simulink model "StateEstimation"  (R2024b)
settings: configuration reference "STM32H7_Config" (kept outside this file)
undefined symbols (not defined in the file): aCamberStaticFL, aCamberStaticFR, aCamberStaticRL, aCamberStaticRR, aCasterFront, AFrontalArea, aKPIFront, aRollGradient, aToeFL, aToeFR, aToeRL, aToeRR, DAirDensity, FTyreVerticalStaticFL, FTyreVerticalStaticFR, FTyreVerticalStaticRL, FTyreVerticalStaticRR, KWheelRateFront, KWheelRateRear, lFrontDistanceCG, lRearDistanceCG, lTrackWidth, lVSALLatFront, lVSALLatRear, lWheelbase, mCarMass, rAckermann, rCL, rCoP, rLLTD, zCoGHeight
libraries: simulink x4
settings Model: DataDictionary=Master_Dictionary.sldd  EnableAccessToBaseWorkspace=off  Creator=torni  LastModifiedBy=Will
settings ConfigSetRef: SourceName=STM32H7_Config

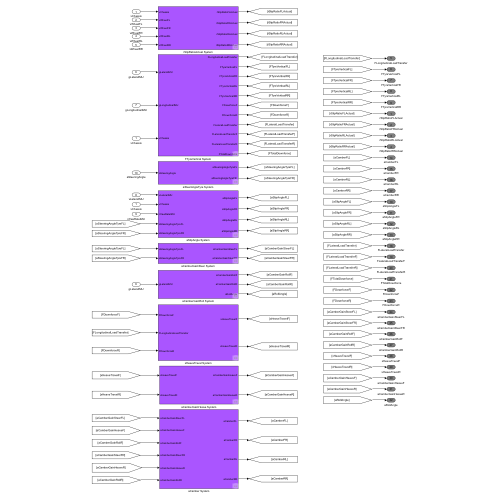
[thumbnail: Simulink's stored preview of the top-level diagram]
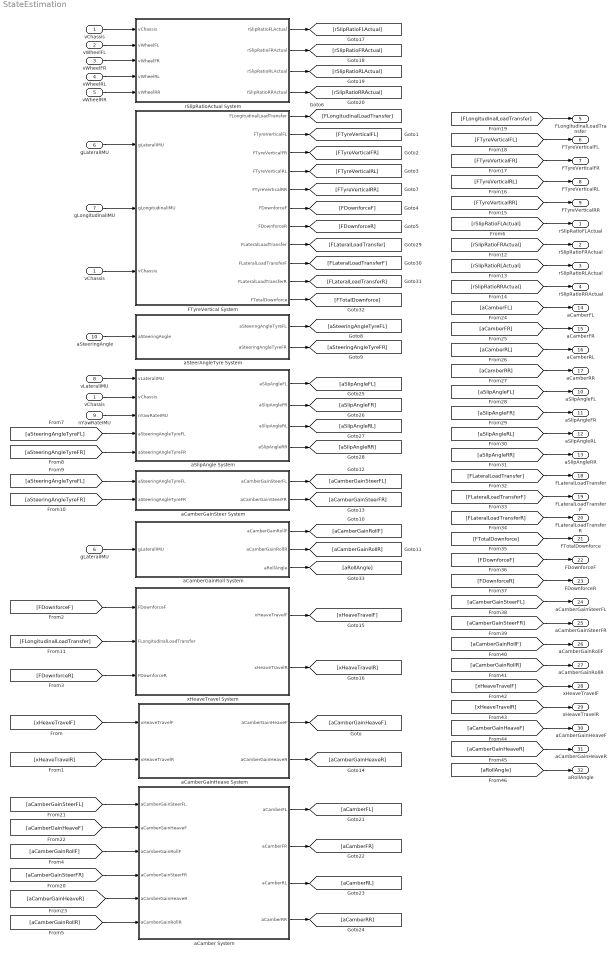
== system StateEstimation ==
  vChassis : Inport
  "vWheelFL " : Inport  Port=2
  "vWheelFR " : Inport  Port=3
  vWheelRL : Inport  Port=4
  vWheelRR : Inport  Port=5
  gLateralIMU : Inport  Port=6  OutDataTypeStr=double
  gLongitudinalIMU : Inport  Port=7  OutDataTypeStr=double
  vLateralIMU : Inport  Port=8
  nYawRateIMU : Inport  Port=9
  "aSteeringAngle " : Inport  Port=10
  FTyreVertical System : Subsystem
  aCamber System : Subsystem
  aCamberGainHeave System : Subsystem
  aCamberGainRoll System : Subsystem
  aCamberGainSteer System : Subsystem
  aSlipAngle System : Subsystem
  aSteerAngleTyre System : Subsystem
  "gLateralIMU " : InportShadow  Port=6  OutDataTypeStr=double
  rSlipRatioActual System : Subsystem
  "vChassis " : InportShadow
  "vChassis " : InportShadow
  xHeaveTravel System : Subsystem
  rSlipRatioFLActual : Outport  VectorParamsAs1DForOutWhenUnconnected=off
  rSlipRatioFRActual : Outport  Port=2  VectorParamsAs1DForOutWhenUnconnected=off
  rSlipRatioRLActual : Outport  Port=3  VectorParamsAs1DForOutWhenUnconnected=off
  rSlipRatioRRActual : Outport  Port=4  VectorParamsAs1DForOutWhenUnconnected=off
  FLongitudinalLoadTransfer : Outport  Port=5  OutDataTypeStr=double  VectorParamsAs1DForOutWhenUnconnected=off
  FTyreVerticalFL : Outport  Port=6  OutDataTypeStr=double  VectorParamsAs1DForOutWhenUnconnected=off
  FTyreVerticalFR : Outport  Port=7  OutDataTypeStr=double  VectorParamsAs1DForOutWhenUnconnected=off
  FTyreVerticalRL : Outport  Port=8  OutDataTypeStr=double  VectorParamsAs1DForOutWhenUnconnected=off
  FTyreVerticalRR : Outport  Port=9  OutDataTypeStr=double  VectorParamsAs1DForOutWhenUnconnected=off
  aSlipAngleFL : Outport  Port=10  VectorParamsAs1DForOutWhenUnconnected=off
  aSlipAngleFR : Outport  Port=11  VectorParamsAs1DForOutWhenUnconnected=off
  aSlipAngleRL : Outport  Port=12  VectorParamsAs1DForOutWhenUnconnected=off
  aSlipAngleRR : Outport  Port=13  VectorParamsAs1DForOutWhenUnconnected=off
  "aCamberFL " : Outport  Port=14  VectorParamsAs1DForOutWhenUnconnected=off
  aCamberFR : Outport  Port=15  VectorParamsAs1DForOutWhenUnconnected=off
  aCamberRL : Outport  Port=16  VectorParamsAs1DForOutWhenUnconnected=off
  aCamberRR : Outport  Port=17  VectorParamsAs1DForOutWhenUnconnected=off
  FLateralLoadTransfer : Outport  Port=18  OutDataTypeStr=double  VectorParamsAs1DForOutWhenUnconnected=off
  FLateralLoadTransferF : Outport  Port=19  OutDataTypeStr=double  VectorParamsAs1DForOutWhenUnconnected=off
  FLateralLoadTransferR : Outport  Port=20  OutDataTypeStr=double  VectorParamsAs1DForOutWhenUnconnected=off
  FTotalDownforce : Outport  Port=21  OutDataTypeStr=double  VectorParamsAs1DForOutWhenUnconnected=off
  FDownforceF : Outport  Port=22  OutDataTypeStr=double  VectorParamsAs1DForOutWhenUnconnected=off
  FDownforceR : Outport  Port=23  OutDataTypeStr=double  VectorParamsAs1DForOutWhenUnconnected=off
  aCamberGainSteerFL : Outport  Port=24  OutDataTypeStr=double  VectorParamsAs1DForOutWhenUnconnected=off
  aCamberGainSteerFR : Outport  Port=25  OutDataTypeStr=double  VectorParamsAs1DForOutWhenUnconnected=off
  aCamberGainRollF : Outport  Port=26  OutDataTypeStr=double  VectorParamsAs1DForOutWhenUnconnected=off
  aCamberGainRollR : Outport  Port=27  OutDataTypeStr=double  VectorParamsAs1DForOutWhenUnconnected=off
  xHeaveTravelF : Outport  Port=28  OutDataTypeStr=double  VectorParamsAs1DForOutWhenUnconnected=off
  xHeaveTravelR : Outport  Port=29  OutDataTypeStr=double  VectorParamsAs1DForOutWhenUnconnected=off
  aCamberGainHeaveF : Outport  Port=30  OutDataTypeStr=double  VectorParamsAs1DForOutWhenUnconnected=off
  aCamberGainHeaveR : Outport  Port=31  OutDataTypeStr=double  VectorParamsAs1DForOutWhenUnconnected=off
  aRollAngle : Outport  Port=32  VectorParamsAs1DForOutWhenUnconnected=off
  wires:
  [aCamberGainHeaveR] -> aCamber System/5("aCamberGainHeaveR ")
  [aCamberGainHeaveF] -> aCamber System/2("aCamberGainHeaveF ")
  aSteerAngleTyre System/1(aSteeringAngleTyreFL) -> [aSteeringAngleTyreFL]
  FTyreVertical System/6(FDownforceF) -> [FDownforceF]
  aCamberGainRoll System/1(aCamberGainRollF) -> [aCamberGainRollF]
  [aCamberGainSteerFR] -> aCamber System/4("aCamberGainSteerFR ")
  aCamberGainSteer System/2(aCamberGainSteerFR) -> [aCamberGainSteerFR]
  [FDownforceF] -> xHeaveTravel System/1("FDownforceF ")
  [aCamberGainRollR] -> aCamber System/6("aCamberGainRollR ")
  [aCamberGainSteerFL] -> aCamber System/1("aCamberGainSteerFL ")
  aCamberGainSteer System/1(aCamberGainSteerFL) -> [aCamberGainSteerFL]
  [FDownforceR] -> xHeaveTravel System/3("FDownforceR ")
  [aSteeringAngleTyreFL] -> aCamberGainSteer System/1(aSteeringAngleTyreFL)
  [FLongitudinalLoadTransfer] -> xHeaveTravel System/2(FLongitudinalLoadTransfer)
  [FTyreVerticalFL] -> FTyreVerticalFL/1
  [FTyreVerticalRR] -> FTyreVerticalRR/1
  "vChassis "/1 -> FTyreVertical System/3(vChassis)
  nYawRateIMU/1 -> aSlipAngle System/3("nYawRateIMU ")
  [FTyreVerticalFR] -> FTyreVerticalFR/1
  gLateralIMU/1 -> FTyreVertical System/1(gLateralIMU)
  aCamberGainRoll System/2(aCamberGainRollR) -> [aCamberGainRollR]
  FTyreVertical System/5(FTyreVerticalRR) -> [FTyreVerticalRR]
  FTyreVertical System/7(FDownforceR) -> [FDownforceR]
  vLateralIMU/1 -> aSlipAngle System/1(vLateralIMU)
  [aSteeringAngleTyreFR] -> aCamberGainSteer System/2(aSteeringAngleTyreFR)
  FTyreVertical System/1(FLongitudinalLoadTransfer) -> [FLongitudinalLoadTransfer]
  FTyreVertical System/3(FTyreVerticalFR) -> [FTyreVerticalFR]
  FTyreVertical System/4(FTyreVerticalRL) -> [FTyreVerticalRL]
  [aSteeringAngleTyreFL] -> aSlipAngle System/4(aSteeringAngleTyreFL)
  "aSteeringAngle "/1 -> aSteerAngleTyre System/1("aSteeringAngle ")
  [FLongitudinalLoadTransfer] -> FLongitudinalLoadTransfer/1
  aSteerAngleTyre System/2("aSteeringAngleTyreFR ") -> [aSteeringAngleTyreFR]
  "gLateralIMU "/1 -> aCamberGainRoll System/1("gLateralIMU ")
  FTyreVertical System/2(FTyreVerticalFL) -> [FTyreVerticalFL]
  [FTyreVerticalRL] -> FTyreVerticalRL/1
  gLongitudinalIMU/1 -> FTyreVertical System/2(gLongitudinalIMU)
  [aCamberGainRollF] -> aCamber System/3("aCamberGainRollF ")
  [aSteeringAngleTyreFR] -> aSlipAngle System/5(aSteeringAngleTyreFR)
  "vChassis "/1 -> aSlipAngle System/2(vChassis)
  xHeaveTravel System/1(xHeaveTravelF) -> [xHeaveTravelF]
  xHeaveTravel System/2(xHeaveTravelR) -> [xHeaveTravelR]
  rSlipRatioActual System/4(rSlipRatioRRActual) -> [rSlipRatioRRActual]
  rSlipRatioActual System/3(rSlipRatioRLActual) -> [rSlipRatioRLActual]
  rSlipRatioActual System/2(rSlipRatioFRActual) -> [rSlipRatioFRActual]
  rSlipRatioActual System/1(rSlipRatioFLActual) -> [rSlipRatioFLActual]
  [rSlipRatioFLActual] -> rSlipRatioFLActual/1
  [rSlipRatioRRActual] -> rSlipRatioRRActual/1
  [rSlipRatioRLActual] -> rSlipRatioRLActual/1
  [rSlipRatioFRActual] -> rSlipRatioFRActual/1
  aCamber System/1("aCamberFL ") -> [aCamberFL]
  aCamber System/2(aCamberFR) -> [aCamberFR]
  aCamber System/3(aCamberRL) -> [aCamberRL]
  aCamber System/4(aCamberRR) -> [aCamberRR]
  [aCamberFL] -> "aCamberFL "/1
  [aCamberFR] -> aCamberFR/1
  [aCamberRL] -> aCamberRL/1
  [aCamberRR] -> aCamberRR/1
  aSlipAngle System/1(aSlipAngleFL) -> [aSlipAngleFL]
  aSlipAngle System/2(aSlipAngleFR) -> [aSlipAngleFR]
  aSlipAngle System/3(aSlipAngleRL) -> [aSlipAngleRL]
  aSlipAngle System/4(aSlipAngleRR) -> [aSlipAngleRR]
  [aSlipAngleFL] -> aSlipAngleFL/1
  [aSlipAngleFR] -> aSlipAngleFR/1
  [aSlipAngleRL] -> aSlipAngleRL/1
  [aSlipAngleRR] -> aSlipAngleRR/1
  aCamberGainHeave System/1(aCamberGainHeaveF) -> [aCamberGainHeaveF]
  aCamberGainHeave System/2(aCamberGainHeaveR) -> [aCamberGainHeaveR]
  [xHeaveTravelF] -> aCamberGainHeave System/1("xHeaveTravelF ")
  [xHeaveTravelR] -> aCamberGainHeave System/2(xHeaveTravelR)
  vChassis/1 -> rSlipRatioActual System/1(vChassis)
  "vWheelFL "/1 -> rSlipRatioActual System/2("vWheelFL ")
  "vWheelFR "/1 -> rSlipRatioActual System/3("vWheelFR ")
  vWheelRL/1 -> rSlipRatioActual System/4(vWheelRL)
  vWheelRR/1 -> rSlipRatioActual System/5(vWheelRR)
  [FLateralLoadTransferR] -> FLateralLoadTransferR/1
  [FLateralLoadTransfer] -> FLateralLoadTransfer/1
  FTyreVertical System/8(FLateralLoadTransfer) -> [FLateralLoadTransfer]
  FTyreVertical System/9(FLateralLoadTransferF) -> [FLateralLoadTransferF]
  FTyreVertical System/10(FLateralLoadTransferR) -> [FLateralLoadTransferR]
  FTyreVertical System/11(FTotalDownforce) -> [FTotalDownforce]
  aCamberGainRoll System/3(aRollAngle) -> [aRollAngle]
  [FLateralLoadTransferF] -> FLateralLoadTransferF/1
  [FTotalDownforce] -> FTotalDownforce/1
  [FDownforceF] -> FDownforceF/1
  [FDownforceR] -> FDownforceR/1
  [aCamberGainSteerFL] -> aCamberGainSteerFL/1
  [aCamberGainSteerFR] -> aCamberGainSteerFR/1
  [aCamberGainRollF] -> aCamberGainRollF/1
  [aCamberGainRollR] -> aCamberGainRollR/1
  [xHeaveTravelF] -> xHeaveTravelF/1
  [xHeaveTravelR] -> xHeaveTravelR/1
  [aCamberGainHeaveF] -> aCamberGainHeaveF/1
  [aCamberGainHeaveR] -> aCamberGainHeaveR/1
  [aRollAngle] -> aRollAngle/1

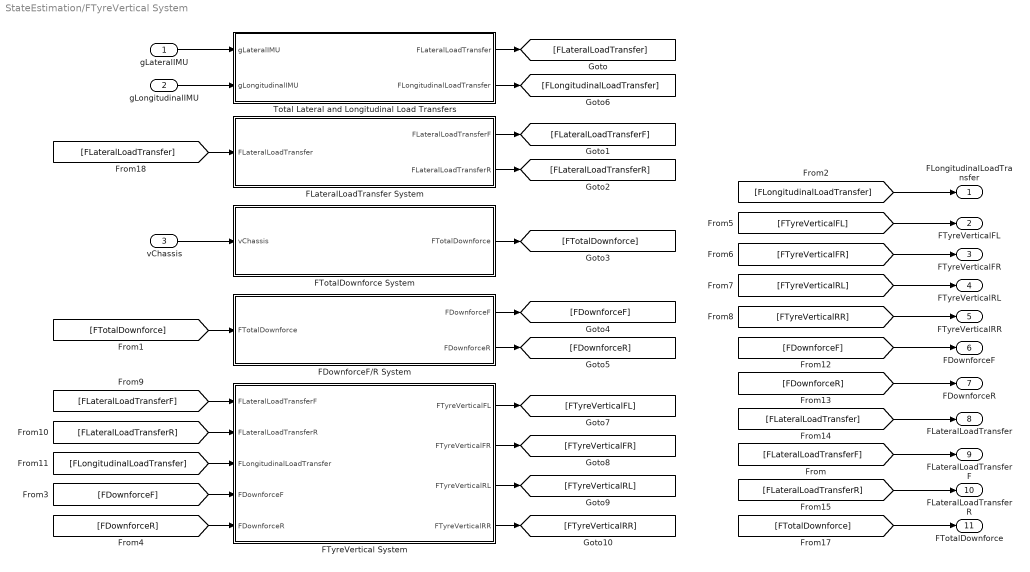
== system StateEstimation/FTyreVertical System ==
  gLateralIMU : Inport  OutDataTypeStr=double
  gLongitudinalIMU : Inport  Port=2  OutDataTypeStr=double
  vChassis : Inport  Port=3
  FDownforceF/R System : Subsystem
  FLateralLoadTransfer System : Subsystem
  FTotalDownforce System : Subsystem
  FTyreVertical System : Subsystem
  Total Lateral and Longitudinal Load Transfers : Subsystem
  FLongitudinalLoadTransfer : Outport  OutDataTypeStr=double  VectorParamsAs1DForOutWhenUnconnected=off
  FTyreVerticalFL : Outport  Port=2  OutDataTypeStr=double  VectorParamsAs1DForOutWhenUnconnected=off
  FTyreVerticalFR : Outport  Port=3  OutDataTypeStr=double  VectorParamsAs1DForOutWhenUnconnected=off
  FTyreVerticalRL : Outport  Port=4  OutDataTypeStr=double  VectorParamsAs1DForOutWhenUnconnected=off
  FTyreVerticalRR : Outport  Port=5  OutDataTypeStr=double  VectorParamsAs1DForOutWhenUnconnected=off
  FDownforceF : Outport  Port=6  OutDataTypeStr=double  VectorParamsAs1DForOutWhenUnconnected=off
  FDownforceR : Outport  Port=7  OutDataTypeStr=double  VectorParamsAs1DForOutWhenUnconnected=off
  FLateralLoadTransfer : Outport  Port=8  OutDataTypeStr=double  VectorParamsAs1DForOutWhenUnconnected=off
  FLateralLoadTransferF : Outport  Port=9  OutDataTypeStr=double  VectorParamsAs1DForOutWhenUnconnected=off
  FLateralLoadTransferR : Outport  Port=10  OutDataTypeStr=double  VectorParamsAs1DForOutWhenUnconnected=off
  FTotalDownforce : Outport  Port=11  OutDataTypeStr=double  VectorParamsAs1DForOutWhenUnconnected=off
  wires:
  [FTotalDownforce] -> FTotalDownforce/1
  FDownforceF/R System/1(FDownforceF) -> [FDownforceF]
  FLateralLoadTransfer System/1(FLateralLoadTransferF) -> [FLateralLoadTransferF]
  [FTotalDownforce] -> FDownforceF/R System/1("FTotalDownforce ")
  [FLateralLoadTransfer] -> FLateralLoadTransfer System/1(FLateralLoadTransfer)
  gLateralIMU/1 -> Total Lateral and Longitudinal Load Transfers/1(gLateralIMU)
  FLateralLoadTransfer System/2(FLateralLoadTransferR) -> [FLateralLoadTransferR]
  vChassis/1 -> FTotalDownforce System/1(vChassis)
  FTotalDownforce System/1(FTotalDownforce) -> [FTotalDownforce]
  Total Lateral and Longitudinal Load Transfers/1(FLateralLoadTransfer) -> [FLateralLoadTransfer]
  FDownforceF/R System/2(FDownforceR) -> [FDownforceR]
  [FLateralLoadTransferF] -> FTyreVertical System/1(FLateralLoadTransferF)
  [FLateralLoadTransferR] -> FTyreVertical System/2(FLateralLoadTransferR)
  [FLongitudinalLoadTransfer] -> FTyreVertical System/3("FLongitudinalLoadTransfer ")
  [FDownforceF] -> FTyreVertical System/4(FDownforceF)
  [FDownforceR] -> FTyreVertical System/5(FDownforceR)
  [FLongitudinalLoadTransfer] -> FLongitudinalLoadTransfer/1
  FTyreVertical System/1(FTyreVerticalFL) -> [FTyreVerticalFL]
  FTyreVertical System/2(FTyreVerticalFR) -> [FTyreVerticalFR]
  FTyreVertical System/3(FTyreVerticalRL) -> [FTyreVerticalRL]
  FTyreVertical System/4(FTyreVerticalRR) -> [FTyreVerticalRR]
  [FTyreVerticalFL] -> FTyreVerticalFL/1
  [FTyreVerticalFR] -> FTyreVerticalFR/1
  [FTyreVerticalRL] -> FTyreVerticalRL/1
  [FTyreVerticalRR] -> FTyreVerticalRR/1
  [FDownforceR] -> FDownforceR/1
  [FDownforceF] -> FDownforceF/1
  gLongitudinalIMU/1 -> Total Lateral and Longitudinal Load Transfers/2(gLongitudinalIMU)
  Total Lateral and Longitudinal Load Transfers/2(FLongitudinalLoadTransfer) -> [FLongitudinalLoadTransfer]
  [FLateralLoadTransfer] -> FLateralLoadTransfer/1
  [FLateralLoadTransferF] -> FLateralLoadTransferF/1
  [FLateralLoadTransferR] -> FLateralLoadTransferR/1

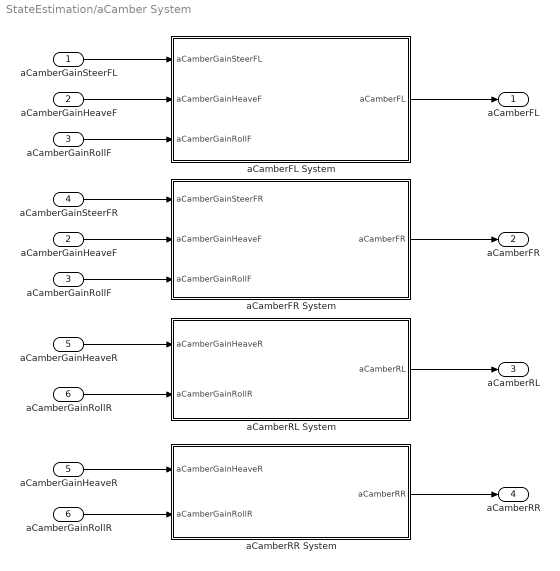
== system StateEstimation/aCamber System ==
  "aCamberGainSteerFL " : Inport
  "aCamberGainHeaveF " : Inport  Port=2
  "aCamberGainRollF " : Inport  Port=3
  "aCamberGainSteerFR " : Inport  Port=4
  "aCamberGainHeaveR " : Inport  Port=5
  "aCamberGainRollR " : Inport  Port=6
  aCamberFL System : Subsystem
  aCamberFR System : Subsystem
  "aCamberGainHeaveF " : InportShadow  Port=2
  "aCamberGainHeaveR " : InportShadow  Port=5
  "aCamberGainRollF " : InportShadow  Port=3
  "aCamberGainRollR " : InportShadow  Port=6
  aCamberRL System : Subsystem
  aCamberRR System : Subsystem
  "aCamberFL " : Outport  VectorParamsAs1DForOutWhenUnconnected=off
  aCamberFR : Outport  Port=2  VectorParamsAs1DForOutWhenUnconnected=off
  aCamberRL : Outport  Port=3  VectorParamsAs1DForOutWhenUnconnected=off
  aCamberRR : Outport  Port=4  VectorParamsAs1DForOutWhenUnconnected=off
  wires:
  "aCamberGainSteerFR "/1 -> aCamberFR System/1("aCamberGainSteerFR ")
  "aCamberGainRollR "/1 -> aCamberRR System/2("aCamberGainRollR ")
  aCamberRR System/1(aCamberRR) -> aCamberRR/1
  aCamberFL System/1("aCamberFL ") -> "aCamberFL "/1
  aCamberFR System/1(aCamberFR) -> aCamberFR/1
  "aCamberGainHeaveF "/1 -> aCamberFR System/2(aCamberGainHeaveF)
  "aCamberGainRollF "/1 -> aCamberFR System/3("aCamberGainRollF ")
  aCamberRL System/1(aCamberRL) -> aCamberRL/1
  "aCamberGainRollR "/1 -> aCamberRL System/2("aCamberGainRollR ")
  "aCamberGainHeaveR "/1 -> aCamberRL System/1("aCamberGainHeaveR ")
  "aCamberGainRollF "/1 -> aCamberFL System/3(aCamberGainRollF)
  "aCamberGainSteerFL "/1 -> aCamberFL System/1(aCamberGainSteerFL)
  "aCamberGainHeaveF "/1 -> aCamberFL System/2("aCamberGainHeaveF ")
  "aCamberGainHeaveR "/1 -> aCamberRR System/1("aCamberGainHeaveR ")

== system StateEstimation/aCamberGainHeave System ==
  note: Camber Gain Heave Angle Front = ( atan ( Heave Travel Distance Front / Virtual Swing Arm Length Lateral Front )) * (180/pi)
  note: Camber Gain Heave Angle Rear = ( atan (Heave Travel Distance Rear / Virtual Swing Arm Length Lateral Rear )) * (180/pi)
  "xHeaveTravelF " : Inport
  xHeaveTravelR : Inport  Port=2
  Constant : Constant  Value=lVSALLatFront
  Constant1 : Constant  Value=lVSALLatRear
  Demux : Demux  Outputs=2
  Divide : Product  Inputs=*/
  Gain : Gain  Gain=180/pi
  Mux : Mux  Inputs=2
  Mux1 : Mux  Inputs=2
  Trigonometric Function : Trigonometry  Operator=atan
  aCamberGainHeaveF : Outport  VectorParamsAs1DForOutWhenUnconnected=off
  aCamberGainHeaveR : Outport  Port=2  VectorParamsAs1DForOutWhenUnconnected=off
  wires:
  Trigonometric Function/1 -> Gain/1
  Divide/1 -> Trigonometric Function/1
  Mux/1 -> Divide/1
  Gain/1 -> Demux/1
  xHeaveTravelR/1 -> Mux/2
  "xHeaveTravelF "/1 -> Mux/1
  Demux/1 -> aCamberGainHeaveF/1
  Demux/2 -> aCamberGainHeaveR/1
  Constant/1 -> Mux1/1
  Mux1/1 -> Divide/2
  Constant1/1 -> Mux1/2

== system StateEstimation/aCamberGainRoll System ==
  "gLateralIMU " : Inport
  aCamberGainRoll System : Subsystem
  aRollAngle System : Subsystem
  aCamberGainRollF : Outport  VectorParamsAs1DForOutWhenUnconnected=off
  aCamberGainRollR : Outport  Port=2  VectorParamsAs1DForOutWhenUnconnected=off
  aRollAngle : Outport  Port=3  VectorParamsAs1DForOutWhenUnconnected=off
  wires:
  "gLateralIMU "/1 -> aRollAngle System/1("gLateralIMU ")
  [aRollAngle] -> aCamberGainRoll System/1(aRollAngle)
  aCamberGainRoll System/1(aCamberGainRollF) -> aCamberGainRollF/1
  aCamberGainRoll System/2("aCamberGainRollR ") -> aCamberGainRollR/1
  aRollAngle System/1("aRollAngle ") -> aRollAngle/1

== system StateEstimation/aCamberGainSteer System ==
  aSteeringAngleTyreFL : Inport
  aSteeringAngleTyreFR : Inport  Port=2
  aCamberGainSteerFL System : Subsystem
  aCamberGainSteerFR System : Subsystem
  aCamberGainSteerFL : Outport  VectorParamsAs1DForOutWhenUnconnected=off
  aCamberGainSteerFR : Outport  Port=2  VectorParamsAs1DForOutWhenUnconnected=off
  wires:
  aSteeringAngleTyreFR/1 -> aCamberGainSteerFR System/1(aSteeringAngleTyreFR)
  aSteeringAngleTyreFL/1 -> aCamberGainSteerFL System/1(aSteeringAngleTyreFL)
  aCamberGainSteerFL System/1(aCamberGainSteerFL) -> aCamberGainSteerFL/1
  aCamberGainSteerFR System/1(aCamberGainSteerFR) -> aCamberGainSteerFR/1

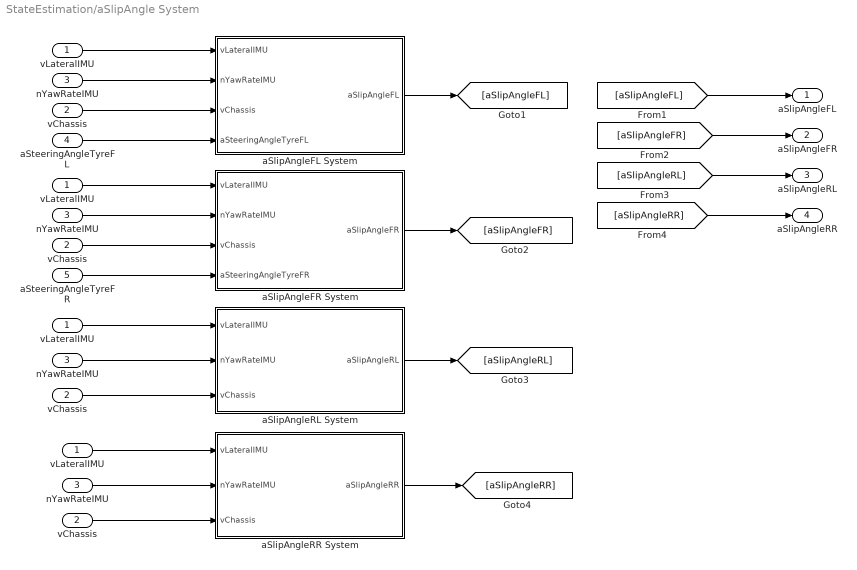
== system StateEstimation/aSlipAngle System ==
  vLateralIMU : Inport
  vChassis : Inport  Port=2
  "nYawRateIMU " : Inport  Port=3
  aSteeringAngleTyreFL : Inport  Port=4
  aSteeringAngleTyreFR : Inport  Port=5
  aSlipAngleFL System : Subsystem
  aSlipAngleFR System : Subsystem
  aSlipAngleRL System : Subsystem
  aSlipAngleRR System : Subsystem
  "nYawRateIMU " : InportShadow  Port=3
  "nYawRateIMU " : InportShadow  Port=3
  "nYawRateIMU " : InportShadow  Port=3
  "vChassis " : InportShadow  Port=2
  "vChassis " : InportShadow  Port=2
  "vChassis " : InportShadow  Port=2
  "vLateralIMU " : InportShadow
  "vLateralIMU " : InportShadow
  "vLateralIMU " : InportShadow
  aSlipAngleFL : Outport  VectorParamsAs1DForOutWhenUnconnected=off
  aSlipAngleFR : Outport  Port=2  VectorParamsAs1DForOutWhenUnconnected=off
  aSlipAngleRL : Outport  Port=3  VectorParamsAs1DForOutWhenUnconnected=off
  aSlipAngleRR : Outport  Port=4  VectorParamsAs1DForOutWhenUnconnected=off
  wires:
  aSlipAngleFR System/1(aSlipAngleFR) -> [aSlipAngleFR]
  "nYawRateIMU "/1 -> aSlipAngleFR System/2(nYawRateIMU)
  [aSlipAngleRR] -> aSlipAngleRR/1
  "nYawRateIMU "/1 -> aSlipAngleFL System/2(nYawRateIMU)
  [aSlipAngleRL] -> aSlipAngleRL/1
  vLateralIMU/1 -> aSlipAngleFL System/1("vLateralIMU ")
  [aSlipAngleFL] -> aSlipAngleFL/1
  "nYawRateIMU "/1 -> aSlipAngleRR System/2("nYawRateIMU  ")
  aSlipAngleRR System/1(aSlipAngleRR) -> [aSlipAngleRR]
  aSteeringAngleTyreFL/1 -> aSlipAngleFL System/4(aSteeringAngleTyreFL)
  "nYawRateIMU "/1 -> aSlipAngleRL System/2("nYawRateIMU ")
  aSteeringAngleTyreFR/1 -> aSlipAngleFR System/4(aSteeringAngleTyreFR)
  [aSlipAngleFR] -> aSlipAngleFR/1
  aSlipAngleFL System/1(aSlipAngleFL) -> [aSlipAngleFL]
  aSlipAngleRL System/1(aSlipAngleRL) -> [aSlipAngleRL]
  vChassis/1 -> aSlipAngleFL System/3("vChassis ")
  "vLateralIMU "/1 -> aSlipAngleFR System/1("vLateralIMU  ")
  "vLateralIMU "/1 -> aSlipAngleRL System/1("vLateralIMU   ")
  "vLateralIMU "/1 -> aSlipAngleRR System/1("vLateralIMU    ")
  "vChassis "/1 -> aSlipAngleFR System/3("vChassis  ")
  "vChassis "/1 -> aSlipAngleRR System/3("vChassis ")
  "vChassis "/1 -> aSlipAngleRL System/3("vChassis   ")

== system StateEstimation/aSteerAngleTyre System ==
  "aSteeringAngle " : Inport
  "aSteeringAngle " : InportShadow
  aSteeringAngleTyreFL System : Subsystem
  aSteeringAngleTyreFR System : Subsystem
  aSteeringAngleTyreFL : Outport  VectorParamsAs1DForOutWhenUnconnected=off
  "aSteeringAngleTyreFR " : Outport  Port=2  VectorParamsAs1DForOutWhenUnconnected=off
  wires:
  aSteeringAngleTyreFL System/1(aSteeringAngleTyreFL) -> aSteeringAngleTyreFL/1
  aSteeringAngleTyreFR System/1("aSteeringAngleTyreFR ") -> "aSteeringAngleTyreFR "/1
  "aSteeringAngle "/1 -> aSteeringAngleTyreFR System/1(aSteeringAngle)
  "aSteeringAngle "/1 -> aSteeringAngleTyreFL System/1(aSteeringAngle)

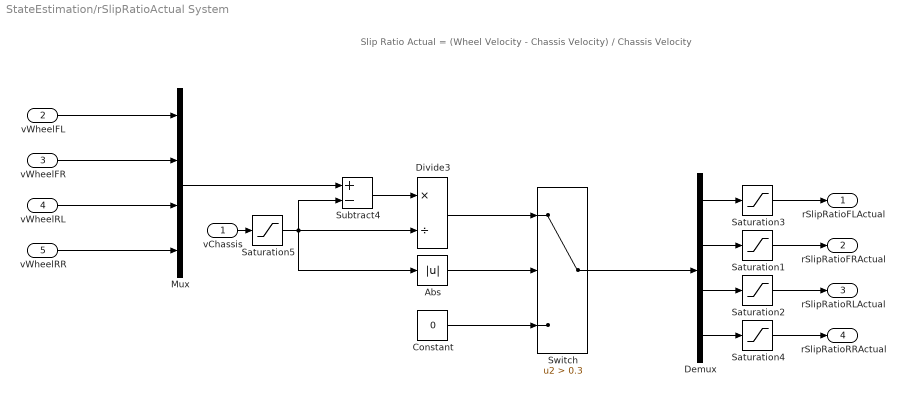
== system StateEstimation/rSlipRatioActual System ==
  note: Slip Ratio Actual = (Wheel Velocity - Chassis Velocity) / Chassis Velocity
  vChassis : Inport
  "vWheelFL " : Inport  Port=2
  "vWheelFR " : Inport  Port=3
  vWheelRL : Inport  Port=4
  vWheelRR : Inport  Port=5
  Abs : Abs  SaturateOnIntegerOverflow=off
  Constant : Constant  Value=0
  Demux : Demux
  Divide3 : Product  Inputs=*/
  Mux : Mux
  Saturation{1..4} (4 alike) : Saturate  UpperLimit=1  LowerLimit=-1
  Saturation5 : Saturate  UpperLimit=35  LowerLimit=0
  Subtract4 : Sum  Inputs=+-
  Switch : Switch  Criteria=u2 > Threshold  Threshold=0.3  SaturateOnIntegerOverflow=off  InputSameDT=off
  rSlipRatioFLActual : Outport  VectorParamsAs1DForOutWhenUnconnected=off
  rSlipRatioFRActual : Outport  Port=2  VectorParamsAs1DForOutWhenUnconnected=off
  rSlipRatioRLActual : Outport  Port=3  VectorParamsAs1DForOutWhenUnconnected=off
  rSlipRatioRRActual : Outport  Port=4  VectorParamsAs1DForOutWhenUnconnected=off
  wires:
  Demux/3 -> Saturation2/1
  Demux/2 -> Saturation1/1
  Abs/1 -> Switch/2
  Subtract4/1 -> Divide3/1
  Demux/1 -> Saturation3/1
  Demux/4 -> Saturation4/1
  Divide3/1 -> Switch/1
  Constant/1 -> Switch/3
  vWheelRR/1 -> Mux/4
  "vWheelFL "/1 -> Mux/1
  Switch/1 -> Demux/1
  vChassis/1 -> Saturation5/1
  "vWheelFR "/1 -> Mux/2
  Mux/1 -> Subtract4/1
  vWheelRL/1 -> Mux/3
  Saturation3/1 -> rSlipRatioFLActual/1
  Saturation1/1 -> rSlipRatioFRActual/1
  Saturation2/1 -> rSlipRatioRLActual/1
  Saturation4/1 -> rSlipRatioRRActual/1
  Saturation5/1 -> Abs/1, Subtract4/2, Divide3/2

== system StateEstimation/xHeaveTravel System ==
  "FDownforceF " : Inport
  FLongitudinalLoadTransfer : Inport  Port=2
  "FDownforceR " : Inport  Port=3
  "FLongitudinalLoadTransfer " : InportShadow  Port=2
  xHeaveTravelF System : Subsystem
  xHeaveTravelR System : Subsystem
  xHeaveTravelF : Outport  VectorParamsAs1DForOutWhenUnconnected=off
  xHeaveTravelR : Outport  Port=2  VectorParamsAs1DForOutWhenUnconnected=off
  wires:
  "FDownforceF "/1 -> xHeaveTravelF System/1("FDownforceF ")
  "FDownforceR "/1 -> xHeaveTravelR System/1("FDownforceR ")
  xHeaveTravelR System/1(xHeaveTravelR) -> xHeaveTravelR/1
  FLongitudinalLoadTransfer/1 -> xHeaveTravelF System/2(FLongitudinalLoadTransfer)
  xHeaveTravelF System/1(xHeaveTravelF) -> xHeaveTravelF/1
  "FLongitudinalLoadTransfer "/1 -> xHeaveTravelR System/2("FLongitudinalLoadTransfer ")

== system StateEstimation/FTyreVertical System/FDownforceF//R System ==
  note: Front Downforce = Total Downforce * CoP
      | Rear Downforce = Total Downforce * (1-CoP)
  "FTotalDownforce " : Inport  OutDataTypeStr=double
  "1 - pCoP " : Gain  Gain=1 - rCoP
  CoP : Gain  Gain=rCoP
  FDownforceF : Outport  OutDataTypeStr=double  VectorParamsAs1DForOutWhenUnconnected=off
  FDownforceR : Outport  Port=2  OutDataTypeStr=double  VectorParamsAs1DForOutWhenUnconnected=off
  wires:
  CoP/1 -> FDownforceF/1
  "FTotalDownforce "/1 -> "1 - pCoP "/1, CoP/1
  "1 - pCoP "/1 -> FDownforceR/1

== system StateEstimation/FTyreVertical System/FLateralLoadTransfer System ==
  note: Front Lateral Load Transfer = Total Lateral Load Transfer * LLTD
  note: Rear Lateral Load Transfer = Total Lateral Load Transfer * (1-LLTD)
  FLateralLoadTransfer : Inport  OutDataTypeStr=double
  1-LLTD : Gain  Gain=1 - rLLTD
  LLTD : Gain  Gain=rLLTD
  FLateralLoadTransferF : Outport  OutDataTypeStr=double  VectorParamsAs1DForOutWhenUnconnected=off
  FLateralLoadTransferR : Outport  Port=2  OutDataTypeStr=double  VectorParamsAs1DForOutWhenUnconnected=off
  wires:
  LLTD/1 -> FLateralLoadTransferF/1
  FLateralLoadTransfer/1 -> 1-LLTD/1, LLTD/1
  1-LLTD/1 -> FLateralLoadTransferR/1

== system StateEstimation/FTyreVertical System/FTotalDownforce System ==
  note: Total Downforce = 0.5 * Air Density * Chassis Velocity ^2 * Frontal area * CL
  vChassis : Inport  OutDataTypeStr=double
  " " : Gain  Gain=0.5
  Air Density : Gain  Gain=DAirDensity
  CL : Gain  Gain=rCL
  Frontal Area : Gain  Gain=AFrontalArea
  Square : Math  Operator=square  SignedPower=on
  FTotalDownforce : Outport  OutDataTypeStr=double  VectorParamsAs1DForOutWhenUnconnected=off
  wires:
  Frontal Area/1 -> CL/1
  " "/1 -> Frontal Area/1
  Air Density/1 -> " "/1
  vChassis/1 -> Square/1
  Square/1 -> Air Density/1
  CL/1 -> FTotalDownforce/1

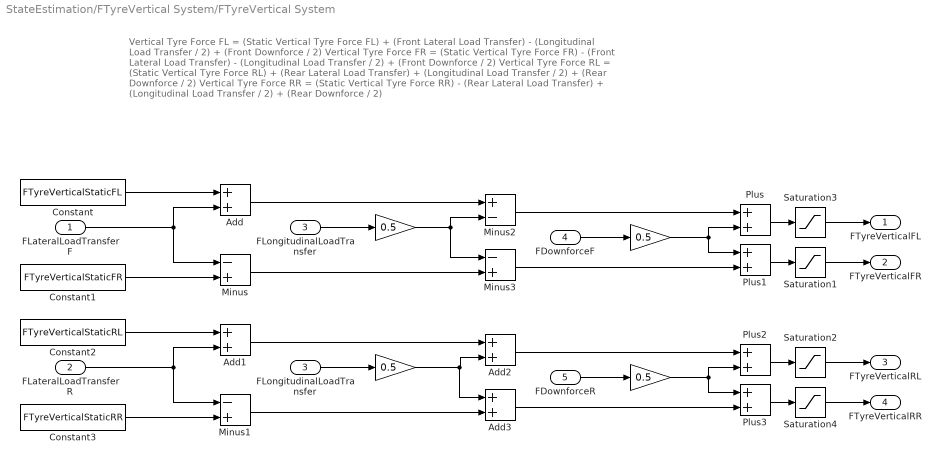
== system StateEstimation/FTyreVertical System/FTyreVertical System ==
  note: Vertical Tyre Force FL = (Static Vertical Tyre Force FL) + (Front Lateral Load Transfer) - (Longitudinal Load Transfer / 2) + (Front Downforce / 2)
      |
      | Vertical Tyre Force FR = (Static Vertical Tyre Force FR) - (Front Lateral Load Transfer) - (Longitudinal Load Transfer / 2) + (Front Downforce / 2)
      |
      | Vertical Tyre Force RL = (Static Vertical Tyre Force RL) + (Rear Lateral Load Transfer) + (Longitudinal Load Transfer / 2) + (Rear Downforce / 2)
      |
      | Vertical Tyre Force RR = (Static Vertical Tyre Force RR) - (Rear Lateral Load Transfer) + (Longitudinal Load Transfer / 2) + (Rear Downforce / 2)
  FLateralLoadTransferF : Inport
  FLateralLoadTransferR : Inport  Port=2
  "FLongitudinalLoadTransfer " : Inport  Port=3
  FDownforceF : Inport  Port=4
  FDownforceR : Inport  Port=5
   {,,,} (4 alike) : Gain  Gain=0.5
  Add{,1..3} (4 alike) : Sum
  Constant : Constant  Value=FTyreVerticalStaticFL
  Constant1 : Constant  Value=FTyreVerticalStaticFR
  Constant2 : Constant  Value=FTyreVerticalStaticRL
  Constant3 : Constant  Value=FTyreVerticalStaticRR
  "FLongitudinalLoadTransfer " : InportShadow  Port=3
  Minus : Sum  Inputs=-+
  Minus1 : Sum  Inputs=-+
  Minus2 : Sum  Inputs=+-
  Minus3 : Sum  Inputs=-+
  Plus{,1..3} (4 alike) : Sum
  Saturation{1..4} (4 alike) : Saturate  UpperLimit=2300  LowerLimit=0
  FTyreVerticalFL : Outport  OutDataTypeStr=double  VectorParamsAs1DForOutWhenUnconnected=off
  FTyreVerticalFR : Outport  Port=2  OutDataTypeStr=double  VectorParamsAs1DForOutWhenUnconnected=off
  FTyreVerticalRL : Outport  Port=3  OutDataTypeStr=double  VectorParamsAs1DForOutWhenUnconnected=off
  FTyreVerticalRR : Outport  Port=4  OutDataTypeStr=double  VectorParamsAs1DForOutWhenUnconnected=off
  wires:
  Minus/1 -> Minus3/2
  "FLongitudinalLoadTransfer "/1 -> " "/1
  FLateralLoadTransferR/1 -> Minus1/1, Add1/2
  FDownforceF/1 -> " "/1
  Minus2/1 -> Plus/1
  " "/1 -> Plus3/1, Plus2/2
  Plus3/1 -> Saturation4/1
  Add2/1 -> Plus2/1
  " "/1 -> Minus3/1, Minus2/2
  Plus2/1 -> Saturation2/1
  " "/1 -> Add3/1, Add2/2
  " "/1 -> Plus1/1, Plus/2
  Constant3/1 -> Minus1/2
  FLateralLoadTransferF/1 -> Minus/1, Add/2
  Constant2/1 -> Add1/1
  FDownforceR/1 -> " "/1
  Add/1 -> Minus2/1
  Plus1/1 -> Saturation1/1
  Constant1/1 -> Minus/2
  Add1/1 -> Add2/1
  Minus3/1 -> Plus1/2
  Minus1/1 -> Add3/2
  Add3/1 -> Plus3/2
  "FLongitudinalLoadTransfer "/1 -> " "/1
  Constant/1 -> Add/1
  Plus/1 -> Saturation3/1
  Saturation3/1 -> FTyreVerticalFL/1
  Saturation1/1 -> FTyreVerticalFR/1
  Saturation2/1 -> FTyreVerticalRL/1
  Saturation4/1 -> FTyreVerticalRR/1

== system StateEstimation/FTyreVertical System/Total Lateral and Longitudinal Load Transfers ==
  note: update values
  note: Lateral Load Transfer = (Lateral Acceleration * Mass * CoG Height) / Trackwidth
  note: Longitudinal Load Transfer = (Longitudinal Acceleration * Mass * CoG Height) / Wheelbase
  gLateralIMU : Inport  OutDataTypeStr=double
  gLongitudinalIMU : Inport  Port=2  OutDataTypeStr=double
  1/Trackwidth : Gain  Gain=1/lTrackWidth
  1/Wheelbase : Gain  Gain=1/lWheelbase
  CoG Height : Gain  Gain=zCoGHeight
  Demux : Demux  Outputs=2
  Mass : Gain  Gain=mCarMass
  Mux : Mux  Inputs=2
  FLateralLoadTransfer : Outport  OutDataTypeStr=double  VectorParamsAs1DForOutWhenUnconnected=off
  FLongitudinalLoadTransfer : Outport  Port=2  OutDataTypeStr=double  VectorParamsAs1DForOutWhenUnconnected=off
  wires:
  Mass/1 -> CoG Height/1
  Mux/1 -> Mass/1
  gLongitudinalIMU/1 -> Mux/2
  gLateralIMU/1 -> Mux/1
  Demux/2 -> 1/Wheelbase/1
  Demux/1 -> 1/Trackwidth/1
  CoG Height/1 -> Demux/1
  1/Wheelbase/1 -> FLongitudinalLoadTransfer/1
  1/Trackwidth/1 -> FLateralLoadTransfer/1

== system StateEstimation/aCamber System/aCamberFL System ==
  note: Camber Angle FL = Static Camber Angle FL + Camber Gain Steer Angle FL - Camber Gain Heave Angle Front + aCamberGainRollFront
  aCamberGainSteerFL : Inport
  "aCamberGainHeaveF " : Inport  Port=2
  aCamberGainRollF : Inport  Port=3
  Add : Sum
  Add1 : Sum
  Constant : Constant  Value=aCamberStaticFL
  Saturation3 : Saturate  UpperLimit=7  LowerLimit=-7
  Subtract : Sum  Inputs=+-
  "aCamberFL " : Outport  VectorParamsAs1DForOutWhenUnconnected=off
  wires:
  Add1/1 -> Saturation3/1
  "aCamberGainHeaveF "/1 -> Subtract/2
  Add/1 -> Subtract/1
  aCamberGainRollF/1 -> Add1/2
  aCamberGainSteerFL/1 -> Add/2
  Subtract/1 -> Add1/1
  Constant/1 -> Add/1
  Saturation3/1 -> "aCamberFL "/1

== system StateEstimation/aCamber System/aCamberFR System ==
  note: Camber Angle FR = Static Camber Angle FR + Camber Gain Steer Angle FR - Camber Gain Heave Angle Front - Camber Gain Roll Angle Front
  "aCamberGainSteerFR " : Inport
  aCamberGainHeaveF : Inport  Port=2
  "aCamberGainRollF " : Inport  Port=3
  Add : Sum
  Constant : Constant  Value=aCamberStaticFR
  Saturation3 : Saturate  UpperLimit=7  LowerLimit=-7
  Subtract : Sum  Inputs=+-
  Subtract1 : Sum  Inputs=+-
  aCamberFR : Outport  VectorParamsAs1DForOutWhenUnconnected=off
  wires:
  Subtract/1 -> Subtract1/1
  "aCamberGainRollF "/1 -> Subtract1/2
  aCamberGainHeaveF/1 -> Subtract/2
  "aCamberGainSteerFR "/1 -> Add/2
  Constant/1 -> Add/1
  Subtract1/1 -> Saturation3/1
  Add/1 -> Subtract/1
  Saturation3/1 -> aCamberFR/1

== system StateEstimation/aCamber System/aCamberRL System ==
  note: Camber Angle RL = Static Camber Angle RL - Camber Gain Heave Angle Rear + Camber Gain Roll Angle Rear
  "aCamberGainHeaveR " : Inport
  "aCamberGainRollR " : Inport  Port=2
  Add : Sum
  Constant : Constant  Value=aCamberStaticRL
  Saturation3 : Saturate  UpperLimit=7  LowerLimit=-7
  Subtract : Sum  Inputs=+-
  aCamberRL : Outport  VectorParamsAs1DForOutWhenUnconnected=off
  wires:
  "aCamberGainHeaveR "/1 -> Subtract/2
  "aCamberGainRollR "/1 -> Add/2
  Subtract/1 -> Add/1
  Add/1 -> Saturation3/1
  Constant/1 -> Subtract/1
  Saturation3/1 -> aCamberRL/1

== system StateEstimation/aCamber System/aCamberRR System ==
  note: Camber Angle RR = Static Camber Angle RR - Camber Gain Heave Angle Rear - Camber Gain Roll Angle Rear
  "aCamberGainHeaveR " : Inport
  "aCamberGainRollR " : Inport  Port=2
  Constant : Constant  Value=aCamberStaticRR
  Saturation3 : Saturate  UpperLimit=7  LowerLimit=-7
  Subtract : Sum  Inputs=+-
  Subtract1 : Sum  Inputs=+-
  aCamberRR : Outport  VectorParamsAs1DForOutWhenUnconnected=off
  wires:
  "aCamberGainHeaveR "/1 -> Subtract/2
  "aCamberGainRollR "/1 -> Subtract1/2
  Subtract/1 -> Subtract1/1
  Subtract1/1 -> Saturation3/1
  Constant/1 -> Subtract/1
  Saturation3/1 -> aCamberRR/1

== system StateEstimation/aCamberGainRoll System/aCamberGainRoll System ==
  note: Camber Gain Roll Angle Front = Roll Angle * (1 - (Trackwidth / (2 * Virtual Swing Arm Length Lateral Front)))
  note: Camber Gain Roll Angle Rear = Roll Angle * (1 - (Trackwidth / (2 * Virtual Swing Arm Length Lateral Rear)))
  aRollAngle : Inport
  Constant : Constant
  Constant1 : Constant  Value=lVSALLatFront
  Constant2 : Constant  Value=lTrackWidth
  Constant3 : Constant  Value=lVSALLatRear
  Demux : Demux  Outputs=2
  Divide : Product  Inputs=*/
  Gain : Gain  Gain=2
  Multiply : Product
  Mux : Mux  Inputs=2
  Saturation3 : Saturate  UpperLimit=10  LowerLimit=-10
  Subtract : Sum  Inputs=+-
  aCamberGainRollF : Outport  VectorParamsAs1DForOutWhenUnconnected=off
  "aCamberGainRollR " : Outport  Port=2  VectorParamsAs1DForOutWhenUnconnected=off
  wires:
  Subtract/1 -> Multiply/1
  Constant2/1 -> Divide/1
  aRollAngle/1 -> Multiply/2
  Constant/1 -> Subtract/1
  Divide/1 -> Subtract/2
  Gain/1 -> Divide/2
  Constant1/1 -> Mux/1
  Constant3/1 -> Mux/2
  Mux/1 -> Gain/1
  Multiply/1 -> Saturation3/1
  Demux/2 -> "aCamberGainRollR "/1
  Demux/1 -> aCamberGainRollF/1
  Saturation3/1 -> Demux/1

== system StateEstimation/aCamberGainRoll System/aRollAngle System ==
  note: Roll Angle = (Roll Gradient * Lateral Acceleration) / 9.81
  "gLateralIMU " : Inport
  Constant : Constant  Value=9.81
  Constant1 : Constant  Value=aRollGradient
  Divide : Product  Inputs=**
  Multiply : Product  Inputs=*/
  Saturation3 : Saturate  UpperLimit=4  LowerLimit=-4
  "aRollAngle " : Outport  VectorParamsAs1DForOutWhenUnconnected=off
  wires:
  Constant1/1 -> Divide/2
  Multiply/1 -> Saturation3/1
  Constant/1 -> Multiply/2
  "gLateralIMU "/1 -> Divide/1
  Divide/1 -> Multiply/1
  Saturation3/1 -> "aRollAngle "/1

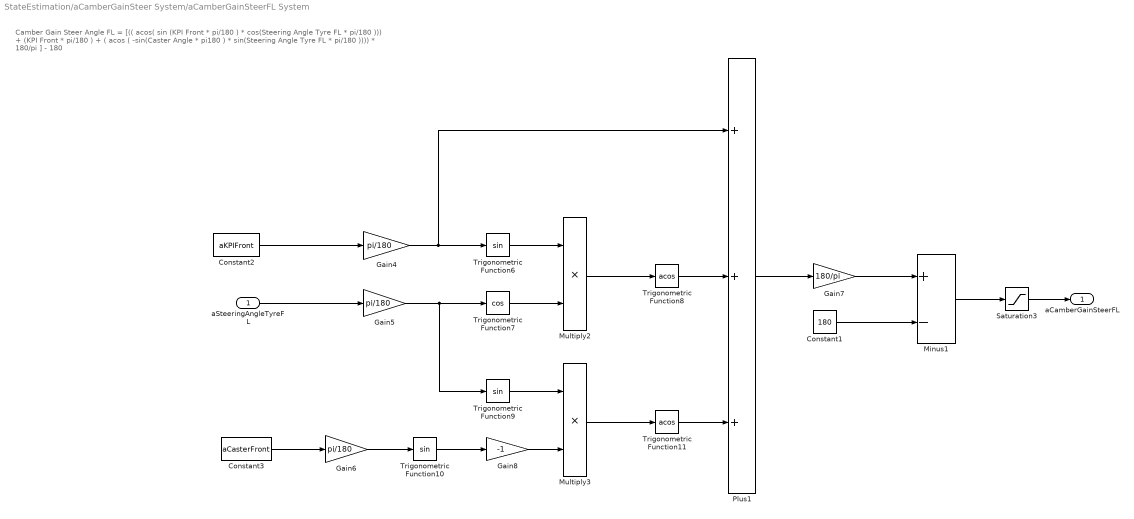
== system StateEstimation/aCamberGainSteer System/aCamberGainSteerFL System ==
  note: Camber Gain Steer Angle FL = [(( acos( sin (KPI Front * pi/180 ) * cos(Steering Angle Tyre FL * pi/180 ))) + (KPI Front * pi/180 ) + ( acos ( -sin(Caster Angle * pi180 ) * sin(Steering Angle Tyre FL * pi/180 )))) * 180/pi ] - 180
  aSteeringAngleTyreFL : Inport
  Constant1 : Constant  Value=180
  Constant2 : Constant  Value=aKPIFront
  Constant3 : Constant  Value=aCasterFront
  Gain4 : Gain  Gain=pi/180
  Gain5 : Gain  Gain=pi/180
  Gain6 : Gain  Gain=pi/180
  Gain7 : Gain  Gain=180/pi
  Gain8 : Gain  Gain=-1
  Minus1 : Sum  Inputs=+-
  Multiply2 : Product
  Multiply3 : Product
  Plus1 : Sum  Inputs=+++
  Saturation3 : Saturate  UpperLimit=5  LowerLimit=-5
  Trigonometric Function10 : Trigonometry
  Trigonometric Function11 : Trigonometry  Operator=acos
  Trigonometric Function6 : Trigonometry
  Trigonometric Function7 : Trigonometry  Operator=cos
  Trigonometric Function8 : Trigonometry  Operator=acos
  Trigonometric Function9 : Trigonometry
  aCamberGainSteerFL : Outport  VectorParamsAs1DForOutWhenUnconnected=off
  wires:
  Gain8/1 -> Multiply3/2
  Trigonometric Function11/1 -> Plus1/3
  Gain7/1 -> Minus1/1
  Gain6/1 -> Trigonometric Function10/1
  Trigonometric Function10/1 -> Gain8/1
  Constant1/1 -> Minus1/2
  Trigonometric Function6/1 -> Multiply2/1
  Plus1/1 -> Gain7/1
  Trigonometric Function8/1 -> Plus1/2
  Minus1/1 -> Saturation3/1
  Multiply3/1 -> Trigonometric Function11/1
  Constant3/1 -> Gain6/1
  Trigonometric Function9/1 -> Multiply3/1
  Multiply2/1 -> Trigonometric Function8/1
  Gain4/1 -> Trigonometric Function6/1, Plus1/1
  Trigonometric Function7/1 -> Multiply2/2
  Gain5/1 -> Trigonometric Function7/1, Trigonometric Function9/1
  Constant2/1 -> Gain4/1
  aSteeringAngleTyreFL/1 -> Gain5/1
  Saturation3/1 -> aCamberGainSteerFL/1

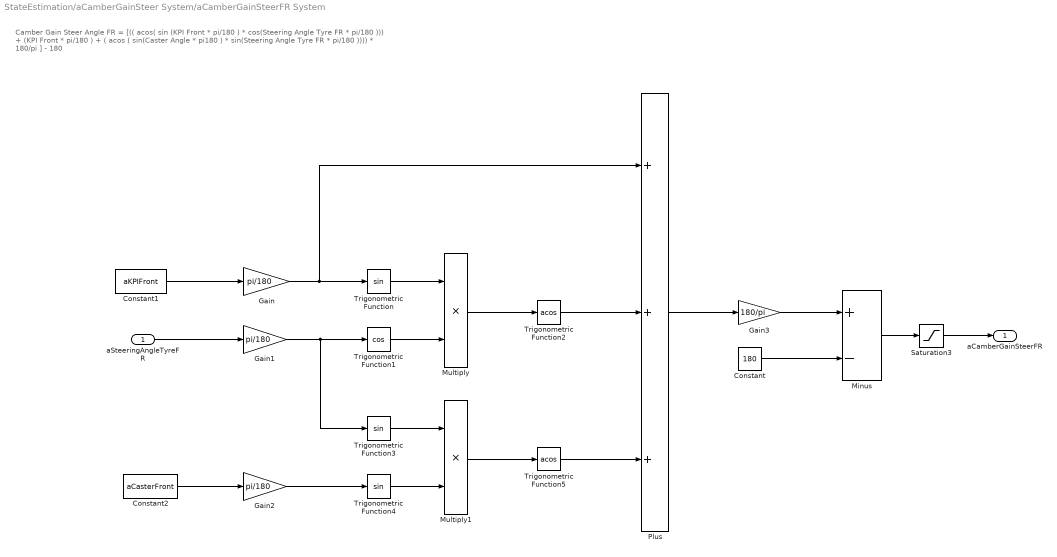
== system StateEstimation/aCamberGainSteer System/aCamberGainSteerFR System ==
  note: Camber Gain Steer Angle FR = [(( acos( sin (KPI Front * pi/180 ) * cos(Steering Angle Tyre FR * pi/180 ))) + (KPI Front * pi/180 ) + ( acos ( sin(Caster Angle * pi180 ) * sin(Steering Angle Tyre FR * pi/180 )))) * 180/pi ] - 180
  aSteeringAngleTyreFR : Inport
  Constant : Constant  Value=180
  Constant1 : Constant  Value=aKPIFront
  Constant2 : Constant  Value=aCasterFront
  Gain : Gain  Gain=pi/180
  Gain1 : Gain  Gain=pi/180
  Gain2 : Gain  Gain=pi/180
  Gain3 : Gain  Gain=180/pi
  Minus : Sum  Inputs=+-
  Multiply : Product
  Multiply1 : Product
  Plus : Sum  Inputs=+++
  Saturation3 : Saturate  UpperLimit=5  LowerLimit=-5
  Trigonometric Function : Trigonometry
  Trigonometric Function1 : Trigonometry  Operator=cos
  Trigonometric Function2 : Trigonometry  Operator=acos
  Trigonometric Function3 : Trigonometry
  Trigonometric Function4 : Trigonometry
  Trigonometric Function5 : Trigonometry  Operator=acos
  aCamberGainSteerFR : Outport  VectorParamsAs1DForOutWhenUnconnected=off
  wires:
  Multiply/1 -> Trigonometric Function2/1
  Gain2/1 -> Trigonometric Function4/1
  Plus/1 -> Gain3/1
  Trigonometric Function1/1 -> Multiply/2
  aSteeringAngleTyreFR/1 -> Gain1/1
  Trigonometric Function5/1 -> Plus/3
  Gain1/1 -> Trigonometric Function3/1, Trigonometric Function1/1
  Gain/1 -> Plus/1, Trigonometric Function/1
  Trigonometric Function3/1 -> Multiply1/1
  Trigonometric Function4/1 -> Multiply1/2
  Multiply1/1 -> Trigonometric Function5/1
  Constant/1 -> Minus/2
  Trigonometric Function2/1 -> Plus/2
  Gain3/1 -> Minus/1
  Minus/1 -> Saturation3/1
  Constant1/1 -> Gain/1
  Trigonometric Function/1 -> Multiply/1
  Constant2/1 -> Gain2/1
  Saturation3/1 -> aCamberGainSteerFR/1

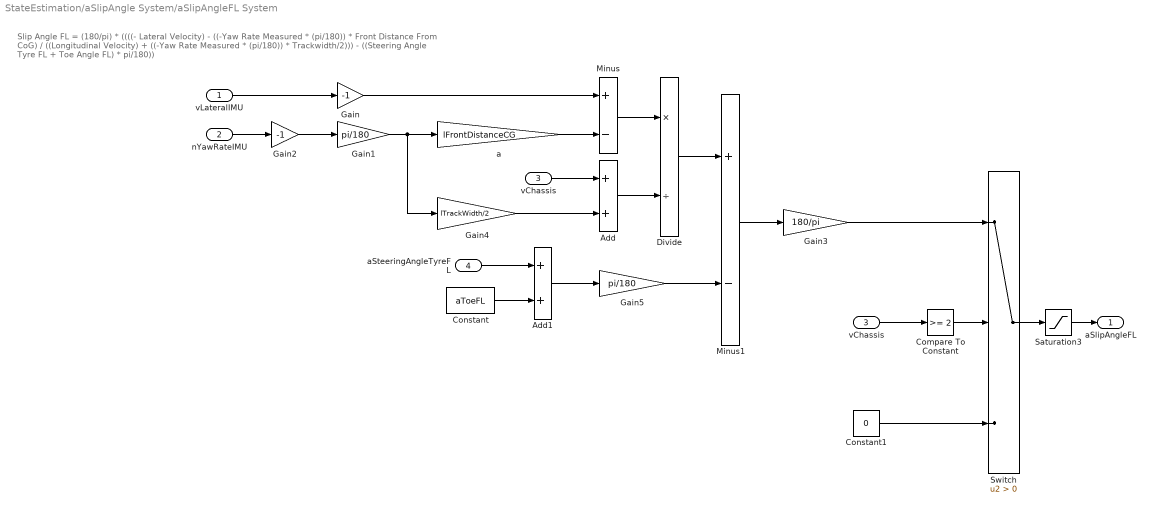
== system StateEstimation/aSlipAngle System/aSlipAngleFL System ==
  note: Slip Angle FL = (180/pi) * ((((- Lateral Velocity) - ((-Yaw Rate Measured * (pi/180)) * Front Distance From CoG) / ((Longitudinal Velocity) + ((-Yaw Rate Measured * (pi/180)) * Trackwidth/2))) - ((Steering Angle Tyre FL + Toe Angle FL) * pi/180))
  "vLateralIMU " : Inport
  nYawRateIMU : Inport  Port=2
  "vChassis " : Inport  Port=3
  aSteeringAngleTyreFL : Inport  Port=4
  Add : Sum
  Add1 : Sum
  Compare To Constant : simulink/Logic and Bit Operations/Compare To Constant  relop=>=  const=2  OutDataTypeStr=boolean
  Constant : Constant  Value=aToeFL
  Constant1 : Constant  Value=0
  Divide : Product  Inputs=*/
  Gain : Gain  Gain=-1
  Gain1 : Gain  Gain=pi/180
  Gain2 : Gain  Gain=-1
  Gain3 : Gain  Gain=180/pi
  Gain4 : Gain  Gain=lTrackWidth/2
  Gain5 : Gain  Gain=pi/180
  Minus : Sum  Inputs=+-
  Minus1 : Sum  Inputs=+-
  Saturation3 : Saturate  UpperLimit=15  LowerLimit=-15
  Switch : Switch  Criteria=u2 > Threshold  SaturateOnIntegerOverflow=off  InputSameDT=off
  a : Gain  Gain=lFrontDistanceCG
  "vChassis " : InportShadow  Port=3
  aSlipAngleFL : Outport  VectorParamsAs1DForOutWhenUnconnected=off
  wires:
  a/1 -> Minus/2
  Gain5/1 -> Minus1/2
  Minus/1 -> Divide/1
  Minus1/1 -> Gain3/1
  nYawRateIMU/1 -> Gain2/1
  "vLateralIMU "/1 -> Gain/1
  Gain4/1 -> Add/2
  Gain1/1 -> a/1, Gain4/1
  aSteeringAngleTyreFL/1 -> Add1/1
  Divide/1 -> Minus1/1
  "vChassis "/1 -> Add/1
  Gain/1 -> Minus/1
  Add1/1 -> Gain5/1
  Add/1 -> Divide/2
  Constant/1 -> Add1/2
  Saturation3/1 -> aSlipAngleFL/1
  "vChassis "/1 -> Compare To Constant/1
  Gain3/1 -> Switch/1
  Switch/1 -> Saturation3/1
  Compare To Constant/1 -> Switch/2
  Constant1/1 -> Switch/3
  Gain2/1 -> Gain1/1

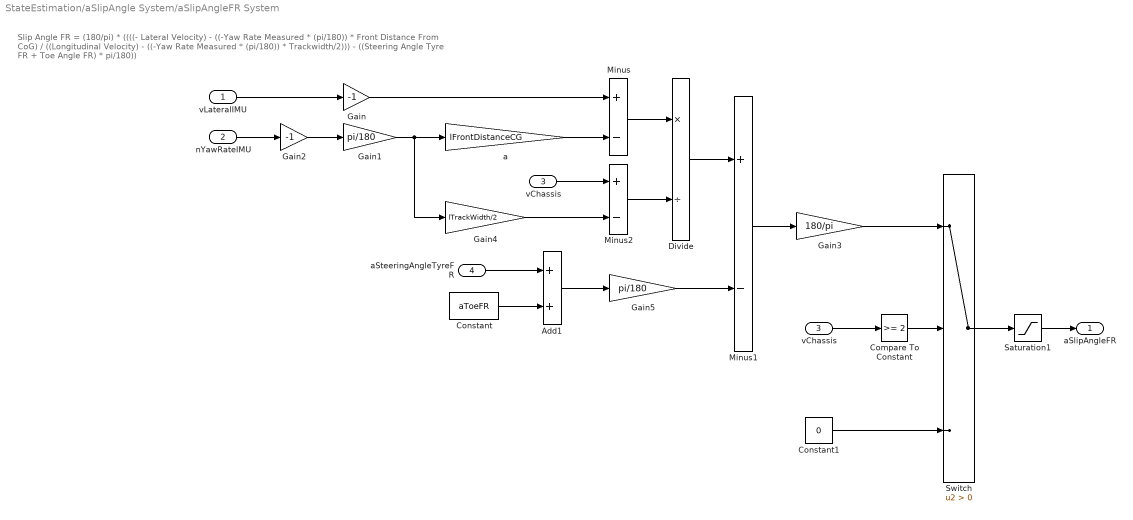
== system StateEstimation/aSlipAngle System/aSlipAngleFR System ==
  note: Slip Angle FR = (180/pi) * ((((- Lateral Velocity) - ((-Yaw Rate Measured * (pi/180)) * Front Distance From CoG) / ((Longitudinal Velocity) - ((-Yaw Rate Measured * (pi/180)) * Trackwidth/2))) - ((Steering Angle Tyre FR + Toe Angle FR) * pi/180))
  "vLateralIMU  " : Inport
  nYawRateIMU : Inport  Port=2
  "vChassis  " : Inport  Port=3
  aSteeringAngleTyreFR : Inport  Port=4
  Add1 : Sum
  Compare To Constant : simulink/Logic and Bit Operations/Compare To Constant  relop=>=  const=2  OutDataTypeStr=boolean
  Constant : Constant  Value=aToeFR
  Constant1 : Constant  Value=0
  Divide : Product  Inputs=*/
  Gain : Gain  Gain=-1
  Gain1 : Gain  Gain=pi/180
  Gain2 : Gain  Gain=-1
  Gain3 : Gain  Gain=180/pi
  Gain4 : Gain  Gain=lTrackWidth/2
  Gain5 : Gain  Gain=pi/180
  Minus : Sum  Inputs=+-
  Minus1 : Sum  Inputs=+-
  Minus2 : Sum  Inputs=+-
  Saturation1 : Saturate  UpperLimit=15  LowerLimit=-15
  Switch : Switch  Criteria=u2 > Threshold  SaturateOnIntegerOverflow=off  InputSameDT=off
  a : Gain  Gain=lFrontDistanceCG
  "vChassis " : InportShadow  Port=3
  aSlipAngleFR : Outport  VectorParamsAs1DForOutWhenUnconnected=off
  wires:
  "vLateralIMU  "/1 -> Gain/1
  Minus2/1 -> Divide/2
  aSteeringAngleTyreFR/1 -> Add1/1
  Gain4/1 -> Minus2/2
  "vChassis  "/1 -> Minus2/1
  Minus/1 -> Divide/1
  Minus1/1 -> Gain3/1
  Gain1/1 -> a/1, Gain4/1
  Add1/1 -> Gain5/1
  Divide/1 -> Minus1/1
  Gain5/1 -> Minus1/2
  a/1 -> Minus/2
  Gain/1 -> Minus/1
  nYawRateIMU/1 -> Gain2/1
  Constant/1 -> Add1/2
  Saturation1/1 -> aSlipAngleFR/1
  Compare To Constant/1 -> Switch/2
  "vChassis "/1 -> Compare To Constant/1
  Constant1/1 -> Switch/3
  Gain3/1 -> Switch/1
  Switch/1 -> Saturation1/1
  Gain2/1 -> Gain1/1

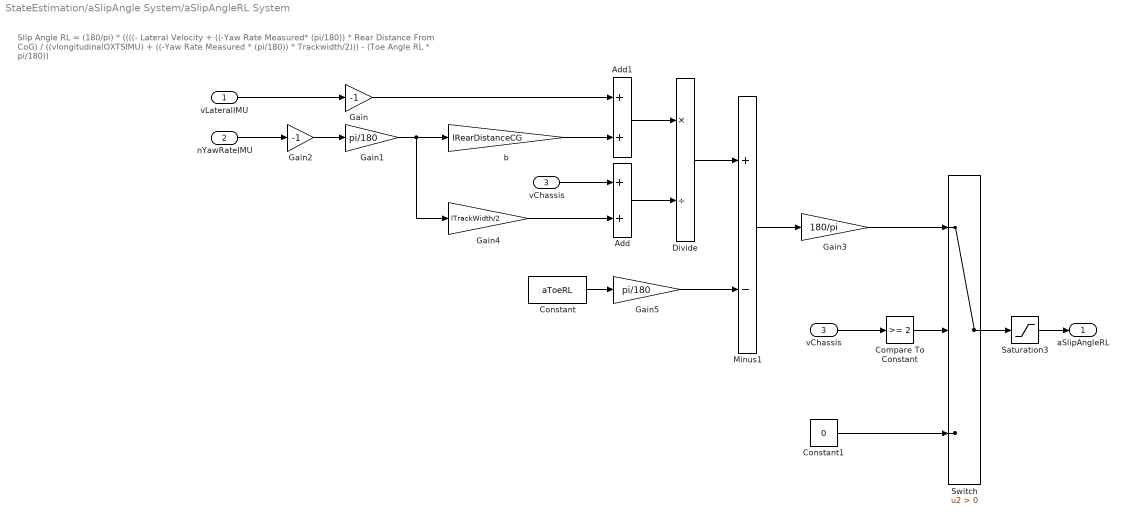
== system StateEstimation/aSlipAngle System/aSlipAngleRL System ==
  note: Slip Angle RL = (180/pi) * ((((- Lateral Velocity + ((-Yaw Rate Measured* (pi/180)) * Rear Distance From CoG) / ((vlongitudinalOXTSIMU) + ((-Yaw Rate Measured * (pi/180)) * Trackwidth/2))) - (Toe Angle RL * pi/180))
  "vLateralIMU   " : Inport
  "nYawRateIMU " : Inport  Port=2
  "vChassis   " : Inport  Port=3
  Add : Sum
  Add1 : Sum
  Compare To Constant : simulink/Logic and Bit Operations/Compare To Constant  relop=>=  const=2  OutDataTypeStr=boolean
  Constant : Constant  Value=aToeRL
  Constant1 : Constant  Value=0
  Divide : Product  Inputs=*/
  Gain : Gain  Gain=-1
  Gain1 : Gain  Gain=pi/180
  Gain2 : Gain  Gain=-1
  Gain3 : Gain  Gain=180/pi
  Gain4 : Gain  Gain=lTrackWidth/2
  Gain5 : Gain  Gain=pi/180
  Minus1 : Sum  Inputs=+-
  Saturation3 : Saturate  UpperLimit=15  LowerLimit=-15
  Switch : Switch  Criteria=u2 > Threshold  SaturateOnIntegerOverflow=off  InputSameDT=off
  b : Gain  Gain=lRearDistanceCG
  "vChassis " : InportShadow  Port=3
  aSlipAngleRL : Outport  VectorParamsAs1DForOutWhenUnconnected=off
  wires:
  Gain1/1 -> b/1, Gain4/1
  Add/1 -> Divide/2
  Gain4/1 -> Add/2
  Divide/1 -> Minus1/1
  Add1/1 -> Divide/1
  "vChassis   "/1 -> Add/1
  Gain5/1 -> Minus1/2
  "vLateralIMU   "/1 -> Gain/1
  Minus1/1 -> Gain3/1
  "nYawRateIMU "/1 -> Gain2/1
  Gain/1 -> Add1/1
  b/1 -> Add1/2
  Constant/1 -> Gain5/1
  Saturation3/1 -> aSlipAngleRL/1
  Compare To Constant/1 -> Switch/2
  "vChassis "/1 -> Compare To Constant/1
  Constant1/1 -> Switch/3
  Gain3/1 -> Switch/1
  Switch/1 -> Saturation3/1
  Gain2/1 -> Gain1/1

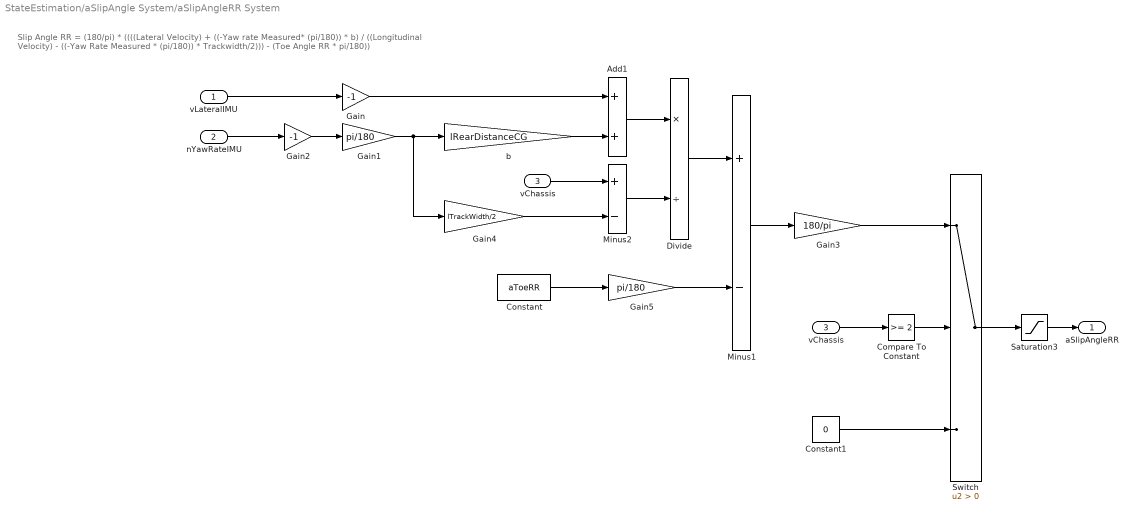
== system StateEstimation/aSlipAngle System/aSlipAngleRR System ==
  note: Slip Angle RR = (180/pi) * ((((Lateral Velocity) + ((-Yaw rate Measured* (pi/180)) * b) / ((Longitudinal Velocity) - ((-Yaw Rate Measured * (pi/180)) * Trackwidth/2))) - (Toe Angle RR * pi/180))
  "vLateralIMU    " : Inport
  "nYawRateIMU  " : Inport  Port=2
  "vChassis " : Inport  Port=3
  Add1 : Sum
  Compare To Constant : simulink/Logic and Bit Operations/Compare To Constant  relop=>=  const=2  OutDataTypeStr=boolean
  Constant : Constant  Value=aToeRR
  Constant1 : Constant  Value=0
  Divide : Product  Inputs=*/
  Gain : Gain  Gain=-1
  Gain1 : Gain  Gain=pi/180
  Gain2 : Gain  Gain=-1
  Gain3 : Gain  Gain=180/pi
  Gain4 : Gain  Gain=lTrackWidth/2
  Gain5 : Gain  Gain=pi/180
  Minus1 : Sum  Inputs=+-
  Minus2 : Sum  Inputs=+-
  Saturation3 : Saturate  UpperLimit=15  LowerLimit=-15
  Switch : Switch  Criteria=u2 > Threshold  SaturateOnIntegerOverflow=off  InputSameDT=off
  b : Gain  Gain=lRearDistanceCG
  "vChassis " : InportShadow  Port=3
  aSlipAngleRR : Outport  VectorParamsAs1DForOutWhenUnconnected=off
  wires:
  Gain5/1 -> Minus1/2
  Add1/1 -> Divide/1
  "vLateralIMU    "/1 -> Gain/1
  "nYawRateIMU  "/1 -> Gain2/1
  "vChassis "/1 -> Minus2/1
  Gain/1 -> Add1/1
  Gain1/1 -> b/1, Gain4/1
  Gain4/1 -> Minus2/2
  Minus1/1 -> Gain3/1
  Minus2/1 -> Divide/2
  Constant/1 -> Gain5/1
  b/1 -> Add1/2
  Divide/1 -> Minus1/1
  Saturation3/1 -> aSlipAngleRR/1
  Compare To Constant/1 -> Switch/2
  "vChassis "/1 -> Compare To Constant/1
  Constant1/1 -> Switch/3
  Gain3/1 -> Switch/1
  Switch/1 -> Saturation3/1
  Gain2/1 -> Gain1/1

== system StateEstimation/aSteerAngleTyre System/aSteeringAngleTyreFL System ==
  note: If steering angle is positive Steering Angle Tyre FL = (200 * Steering Angle) / (200 - Ackermann)
      | If steering angle is negative Steering Angle Tyre FL = Steering Angle * (200 - (2 * Ackermann)) / (200 - Ackermann)
  aSteeringAngle : Inport
  Constant : Constant  Value=200
  Constant1 : Constant  Value=rAckermann
  Constant2 : Constant  Value=200
  Constant3 : Constant  Value=rAckermann
  Divide : Product  Inputs=*/
  Divide1 : Product  Inputs=*/
  Gain : Gain  Gain=2
  Multiply : Product
  Multiply1 : Product
  Subtract : Sum  Inputs=+-
  Subtract1 : Sum  Inputs=+-
  Subtract2 : Sum  Inputs=+-
  Switch : Switch  Criteria=u2 > Threshold  SaturateOnIntegerOverflow=off  InputSameDT=off
  "aSteeringAngle " : InportShadow
  "aSteeringAngle " : InportShadow
  aSteeringAngleTyreFL : Outport  VectorParamsAs1DForOutWhenUnconnected=off
  wires:
  Constant3/1 -> Subtract2/2, Gain/1
  Gain/1 -> Subtract1/2
  Subtract1/1 -> Multiply1/2
  Subtract2/1 -> Divide/2
  Constant2/1 -> Subtract2/1, Subtract1/1
  Multiply/1 -> Divide1/1
  Subtract/1 -> Divide1/2
  Constant1/1 -> Subtract/2
  Switch/1 -> aSteeringAngleTyreFL/1
  Constant/1 -> Subtract/1, Multiply/2
  Divide1/1 -> Switch/1
  Multiply1/1 -> Divide/1
  aSteeringAngle/1 -> Switch/2
  Divide/1 -> Switch/3
  "aSteeringAngle "/1 -> Multiply1/1
  "aSteeringAngle "/1 -> Multiply/1

== system StateEstimation/aSteerAngleTyre System/aSteeringAngleTyreFR System ==
  note: If steering angle is positive Steering Angle Tyre FR = Steering Angle * (200 - (2 * Ackermann)) / (200 - Ackermann)
      | If steering angle is negative Steering Angle Tyre FR = (200 * Steering Angle) / (200 - Ackermann)
  aSteeringAngle : Inport
  Constant : Constant  Value=200
  Constant1 : Constant  Value=rAckermann
  Constant2 : Constant  Value=200
  Constant3 : Constant  Value=rAckermann
  Divide : Product  Inputs=*/
  Divide1 : Product  Inputs=*/
  Gain : Gain  Gain=2
  Multiply : Product
  Multiply1 : Product
  Subtract : Sum  Inputs=+-
  Subtract1 : Sum  Inputs=+-
  Subtract2 : Sum  Inputs=+-
  Switch : Switch  Criteria=u2 > Threshold  SaturateOnIntegerOverflow=off  InputSameDT=off
  "aSteeringAngle " : InportShadow
  "aSteeringAngle " : InportShadow
  "aSteeringAngleTyreFR " : Outport  VectorParamsAs1DForOutWhenUnconnected=off
  wires:
  Switch/1 -> "aSteeringAngleTyreFR "/1
  Constant3/1 -> Subtract2/2, Gain/1
  Gain/1 -> Subtract1/2
  Subtract1/1 -> Multiply1/2
  Subtract2/1 -> Divide/2
  Constant2/1 -> Subtract2/1, Subtract1/1
  Multiply/1 -> Divide1/1
  Subtract/1 -> Divide1/2
  Constant1/1 -> Subtract/2
  Constant/1 -> Subtract/1, Multiply/2
  Multiply1/1 -> Divide/1
  aSteeringAngle/1 -> Switch/2
  Divide/1 -> Switch/1
  Divide1/1 -> Switch/3
  "aSteeringAngle "/1 -> Multiply1/1
  "aSteeringAngle "/1 -> Multiply/1

== system StateEstimation/xHeaveTravel System/xHeaveTravelF System ==
  note: Heave Travel Distance Front = (Front Downforce - Longitudinal Load Transfer) / (2 * Wheel Rate Front)
  "FDownforceF " : Inport
  FLongitudinalLoadTransfer : Inport  Port=2
  Constant : Constant  Value=KWheelRateFront
  Gain : Gain  Gain=2
  Multiply : Product  Inputs=*/
  Saturation3 : Saturate  UpperLimit=0.03  LowerLimit=-0.03
  Subtract : Sum  Inputs=+-
  xHeaveTravelF : Outport  VectorParamsAs1DForOutWhenUnconnected=off
  wires:
  Multiply/1 -> Saturation3/1
  Subtract/1 -> Multiply/1
  Gain/1 -> Multiply/2
  "FDownforceF "/1 -> Subtract/1
  FLongitudinalLoadTransfer/1 -> Subtract/2
  Constant/1 -> Gain/1
  Saturation3/1 -> xHeaveTravelF/1

== system StateEstimation/xHeaveTravel System/xHeaveTravelR System ==
  note: Heave Travel Distance Rear = (Rear Downforce + Longitudinal Load Transfer) / (2 * Wheel Rate Rear)
  "FDownforceR " : Inport
  "FLongitudinalLoadTransfer " : Inport  Port=2
  Add : Sum
  Constant : Constant  Value=KWheelRateRear
  Gain : Gain  Gain=2
  Multiply : Product  Inputs=*/
  Saturation3 : Saturate  UpperLimit=0.03  LowerLimit=-0.03
  xHeaveTravelR : Outport  VectorParamsAs1DForOutWhenUnconnected=off
  wires:
  "FLongitudinalLoadTransfer "/1 -> Add/2
  "FDownforceR "/1 -> Add/1
  Multiply/1 -> Saturation3/1
  Add/1 -> Multiply/1
  Constant/1 -> Gain/1
  Gain/1 -> Multiply/2
  Saturation3/1 -> xHeaveTravelR/1
